simulink model "integral_windup"  (R2024a)
settings: Solver=VariableStepAuto  StartTime=0.0  StopTime=10.0  RelTol=1e-3
settings Model: Creator=johba  LastModifiedBy=johba

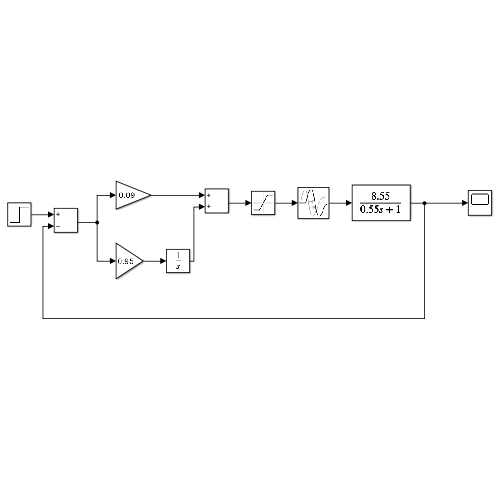
[thumbnail: Simulink's stored preview of the top-level diagram]
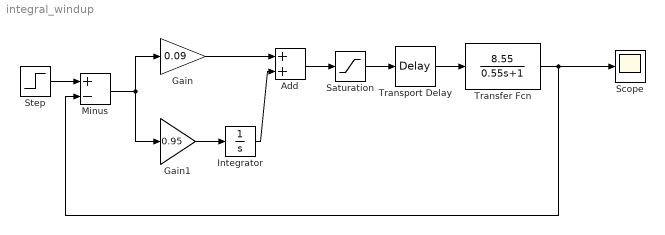
== system integral_windup ==
  Add : Sum
  Gain : Gain  Gain=0.09
  Gain1 : Gain  Gain=0.95
  Integrator : Integrator
  Minus : Sum  Inputs=+-
  Saturation : Saturate  UpperLimit=1.7  LowerLimit=-1.7
  Scope : Scope
  Step : Step  SampleTime=0
  Transfer Fcn : TransferFcn  Numerator=[8.55]  Denominator=[0.55 1]
  Transport Delay : TransportDelay  DelayTime=0.15
  wires:
  Gain1/1 -> Integrator/1
  Gain/1 -> Add/1
  Integrator/1 -> Add/2
  Minus/1 -> Gain1/1, Gain/1
  Add/1 -> Saturation/1
  Saturation/1 -> Transport Delay/1
  Transport Delay/1 -> Transfer Fcn/1
  Step/1 -> Minus/1
  Transfer Fcn/1 -> Minus/2, Scope/1
